simulink model "VLI_OLC_sim"  (R2023a)
settings: Solver=VariableStepAuto  StartTime=0.0  StopTime=1000  RelTol=1e-3
values from neighbouring files (symbols this model uses):
  E = diag([0.95, 0.95, 0.95])    [VLI_OLC_parameter.m]
  J0 = [20, 2, 0.9; 2, 17, 0.5; 0.9, 0.5, 15]    [VLI_OLC_parameter.m]
  k2 = 1    [VLI_OLC_parameter.m]
  k3 = 2    [VLI_OLC_parameter.m]
  Q0 = [-0.2, 0.3, -0.2]    [VLI_OLC_parameter.m]
  Q00 = sqrt(0.83)    [VLI_OLC_parameter.m]
  sig = 1    [VLI_OLC_parameter.m]
  td = 0.01    [VLI_OLC_parameter.m]
  tor = 0.01    [VLI_OLC_parameter.m]
  torque0 = 0.001    [VLI_OLC_parameter.m]
  Tu = 0.03    [VLI_OLC_parameter.m]
  Tv = 0.03    [VLI_OLC_parameter.m]
  w0 = [0, 0, 0]'    [VLI_OLC_parameter.m]
libraries: matrix_library x3, sharedutil x1
settings Model: Creator=bin.lu  LastModifiedBy=bin.lu
settings DataIOCC: ReturnWorkspaceOutputs=off  TimeSaveName=t1

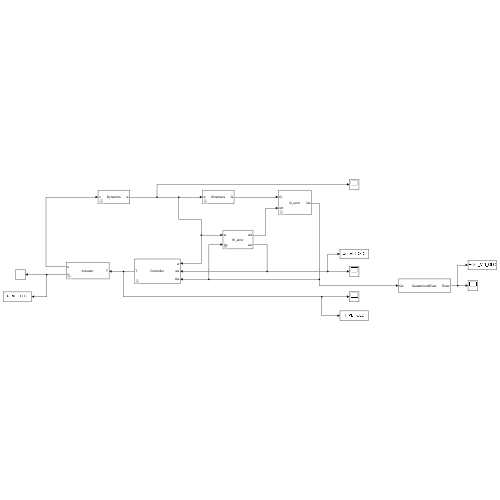
[thumbnail: Simulink's stored preview of the top-level diagram]
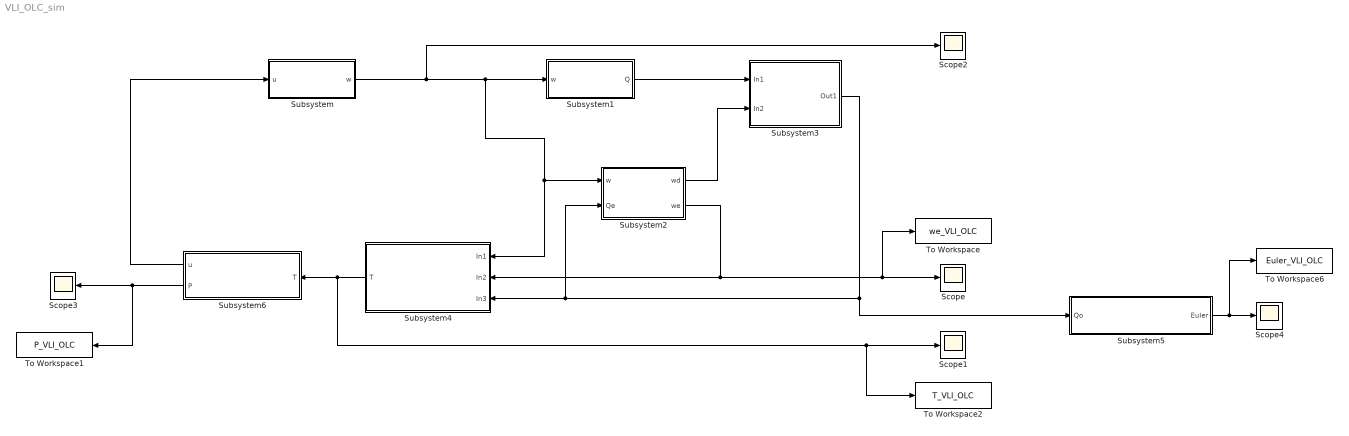
== system VLI_OLC_sim ==
  Scope{,1..4} (5 alike) : Scope
  Subsystem : Subsystem
      mask DialogControl ParameterGroupVar Prompt: 参数
      mask Display:
      | disp('Dynamics');
      | port_label('input', 1, 'u');
      | port_label('output', 1, 'w');
  Subsystem1 : Subsystem
      mask DialogControl ParameterGroupVar Prompt: 参数
      mask Display:
      | disp('Kinemacs');
      | port_label('input', 1, 'w');
      | port_label('output', 1, 'Q');
  Subsystem2 : Subsystem
      mask DialogControl ParameterGroupVar Prompt: 参数
      mask Display:
      | disp('W_error');
      | port_label('input', 1, 'w');
      | port_label('input', 2, 'Qe');
      | port_label('output', 2, 'we');
      | port_label('output', 1, 'wd');
  Subsystem3 : Subsystem
      mask DialogControl ParameterGroupVar Prompt: 参数
      mask Display:
      | disp('Q_error');
      | port_label('input', 1, 'Q');
      | port_label('input', 2, 'wd');
      | port_label('output', 1, 'Qe');
  Subsystem4 : Subsystem
      mask DialogControl ParameterGroupVar Prompt: 参数
      mask Display:
      | disp('Controller');
      | port_label('input', 1, 'w');
      | port_label('input', 2, 'we');
      | port_label('input', 3, 'Qe');
      | port_label('output', 1, 'T');
  Subsystem5 : Subsystem
      mask Display:
      | disp('Quaternion2Euler')
      | port_label('input', 1, 'Qo')
      | port_label('output', 1, 'Euler')
  Subsystem6 : Subsystem
      mask DialogControl ParameterGroupVar Prompt: 参数
      mask Display:
      | disp('Actuator');
      | port_label('input', 1, 'T');
      | port_label('output', 1, 'u');
      | port_label('output', 2, 'P');
  To Workspace : ToWorkspace  VariableName=we_VLI_OLC  SampleTime=-1
      settings: Save2DSignal=2-D array (concatenate along first dimension)
  To Workspace1 : ToWorkspace  VariableName=P_VLI_OLC  SampleTime=0.01
  To Workspace2 : ToWorkspace  VariableName=T_VLI_OLC  SampleTime=-1
      settings: Save2DSignal=2-D array (concatenate along first dimension)
  To Workspace6 : ToWorkspace  VariableName=Euler_VLI_OLC  SampleTime=-1
      settings: Save2DSignal=2-D array (concatenate along first dimension)
  wires:
  Subsystem2/1(wd) -> Subsystem3/2(In2)
  Subsystem3/1(Out1) -> Subsystem5/1(Qo), Subsystem2/2(Qe), Subsystem4/3(In3)
  Subsystem6/2(P) -> To Workspace1/1, Scope3/1
  Subsystem2/2(we) -> Subsystem4/2(In2), To Workspace/1, Scope/1
  Subsystem4/1(T) -> To Workspace2/1, Scope1/1, Subsystem6/1(T)
  Subsystem6/1(u) -> Subsystem/1(u)
  Subsystem1/1(Q) -> Subsystem3/1(In1)
  Subsystem/1(w) -> Subsystem1/1(w), Subsystem4/1(In1), Subsystem2/1(w), Scope2/1
  Subsystem5/1(Euler) -> To Workspace6/1, Scope4/1

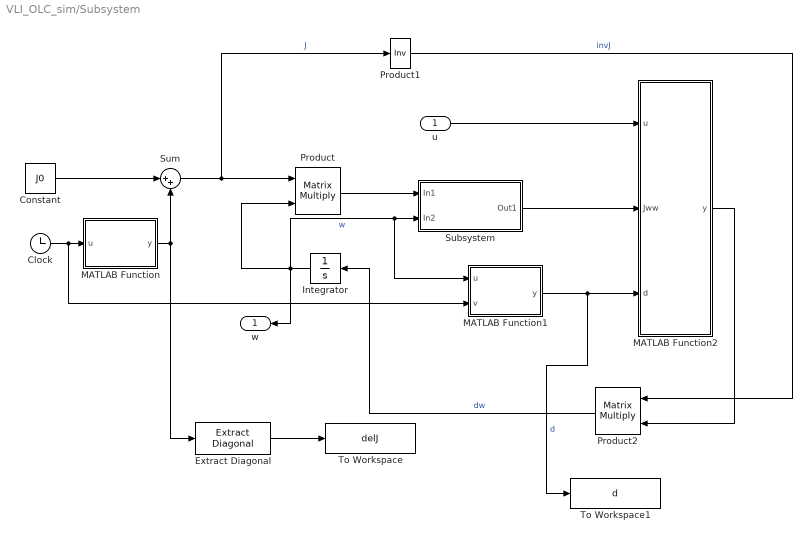
== system VLI_OLC_sim/Subsystem ==
  u : Inport
  Clock : Clock
  Constant : Constant  Value=J0
  Extract Diagonal : matrix_library/Extract Diagonal
      settings: LibrarySourceBlock=|
      | simulink/Matrix
      | Operations/Extract Diagonal
  Integrator : Integrator  InitialCondition=w0
  MATLAB Function : MATLAB Function  TreatAsAtomicUnit=on
  MATLAB Function1 : MATLAB Function  TreatAsAtomicUnit=on
  MATLAB Function2 : MATLAB Function  TreatAsAtomicUnit=on
  Product : Product  Multiplication=Matrix(*)
  Product1 : Product  Inputs=/  Multiplication=Matrix(*)
  Product2 : Product  Multiplication=Matrix(*)
  Subsystem : Subsystem
      mask Display:
      | disp('Cross \nProduct')
      | port_label('input', 1, 'X')
      | port_label('input', 2, 'Y')
      | port_label('output', 1, 'X*Y')
  Sum : Sum  Inputs=|++
  To Workspace : ToWorkspace  VariableName=delJ  SampleTime=-1
      settings: Save2DSignal=2-D array (concatenate along first dimension)
  To Workspace1 : ToWorkspace  VariableName=d  SampleTime=-1
      settings: Save2DSignal=2-D array (concatenate along first dimension)
  w : Outport
  wires:
  MATLAB Function/1(y) -> Extract Diagonal/1, Sum/2
  Constant/1 -> Sum/1
  Clock/1 -> MATLAB Function1/2(v), MATLAB Function/1(u)
  Sum/1 -> Product1/1, Product/1  "J"
  Integrator/1 -> w/1, MATLAB Function1/1(u), Subsystem/2(In2), Product/2  "w"
  Product/1 -> Subsystem/1(In1)
  Subsystem/1(Out1) -> MATLAB Function2/2(Jww)
  Product2/1 -> Integrator/1  "dw"
  MATLAB Function1/1(y) -> To Workspace1/1, MATLAB Function2/3(d)  "d"
  u/1 -> MATLAB Function2/1(u)
  MATLAB Function2/1(y) -> Product2/2
  Product1/1 -> Product2/1  "invJ"
  Extract Diagonal/1 -> To Workspace/1

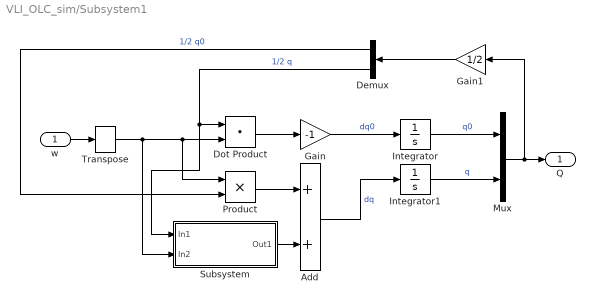
== system VLI_OLC_sim/Subsystem1 ==
  w : Inport
  Add : Sum
  Demux : Demux  Outputs=[1 3]
  Dot Product : DotProduct  OutDataTypeStr=Inherit: Inherit via internal rule
  Gain : Gain  Gain=-1
  Gain1 : Gain  Gain=1/2
  Integrator : Integrator  InitialCondition=Q00
  Integrator1 : Integrator  InitialCondition=Q0
  Mux : Mux  Inputs=[1 3]
  Product : Product
  Subsystem : Subsystem
      mask Display:
      | disp('Cross \nProduct')
      | port_label('input', 1, 'X')
      | port_label('input', 2, 'Y')
      | port_label('output', 1, 'X*Y')
  Transpose : matrix_library/Transpose
  Q : Outport
  wires:
  Dot Product/1 -> Gain/1
  w/1 -> Transpose/1
  Add/1 -> Integrator1/1  "dq"
  Demux/2 -> Subsystem/1(In1), Dot Product/1  "1/2 q"
  Integrator1/1 -> Mux/2  "q"
  Product/1 -> Add/1
  Gain/1 -> Integrator/1  "dq0"
  Integrator/1 -> Mux/1  "q0"
  Mux/1 -> Gain1/1, Q/1
  Gain1/1 -> Demux/1
  Subsystem/1(Out1) -> Add/2
  Demux/1 -> Product/2  "1/2 q0"
  Transpose/1 -> Subsystem/2(In2), Product/1, Dot Product/2

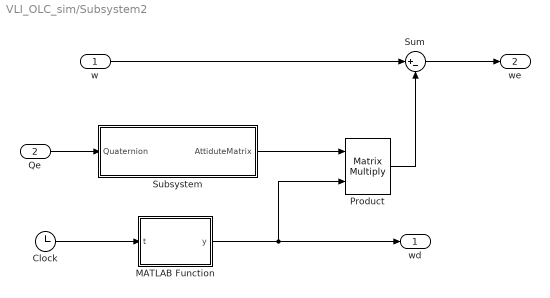
== system VLI_OLC_sim/Subsystem2 ==
  w : Inport
  Qe : Inport  Port=2
  Clock : Clock
  MATLAB Function : MATLAB Function  TreatAsAtomicUnit=on
  Product : Product  Multiplication=Matrix(*)
  Subsystem : Subsystem
      mask Display:
      | disp('Quaternion2 \nAttitudeMatrix')
      | port_label('input', 1, 'Qua')
      | port_label('output', 1, 'Matrix')
  Sum : Sum  Inputs=|+-
  wd : Outport
  we : Outport  Port=2
  wires:
  Qe/1 -> Subsystem/1(Quaternion)
  Clock/1 -> MATLAB Function/1(t)
  Subsystem/1(AttiduteMatrix) -> Product/1
  MATLAB Function/1(y) -> wd/1, Product/2
  w/1 -> Sum/1
  Sum/1 -> we/1
  Product/1 -> Sum/2

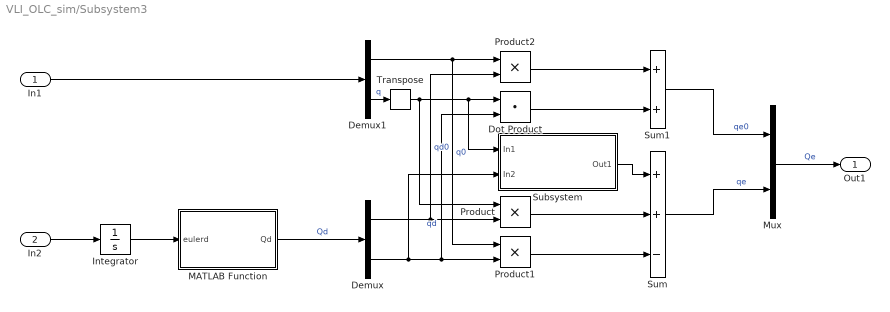
== system VLI_OLC_sim/Subsystem3 ==
  In1 : Inport
  In2 : Inport  Port=2
  Demux : Demux  Outputs=[1 3]
  Demux1 : Demux  Outputs=[1 3]
  Dot Product : DotProduct  OutDataTypeStr=Inherit: Inherit via internal rule
  Integrator : Integrator
  MATLAB Function : MATLAB Function  TreatAsAtomicUnit=on
  Mux : Mux  Inputs=[1 3]
  Product : Product
  Product1 : Product
  Product2 : Product
  Subsystem : Subsystem
      mask Display:
      | disp('Cross \nProduct')
      | port_label('input', 1, 'X')
      | port_label('input', 2, 'Y')
      | port_label('output', 1, 'X*Y')
  Sum : Sum  Inputs=++-
  Sum1 : Sum
  Transpose : matrix_library/Transpose
  Out1 : Outport
  wires:
  In2/1 -> Integrator/1
  Integrator/1 -> MATLAB Function/1(eulerd)
  MATLAB Function/1(Qd) -> Demux/1  "Qd"
  In1/1 -> Demux1/1
  Demux/1 -> Product2/2, Product/2  "qd0"
  Demux1/2 -> Transpose/1  "q"
  Demux/2 -> Subsystem/2(In2), Dot Product/2, Product1/2  "qd"
  Demux1/1 -> Product2/1, Product1/1  "q0"
  Subsystem/1(Out1) -> Sum/1
  Product/1 -> Sum/2
  Product1/1 -> Sum/3
  Product2/1 -> Sum1/1
  Dot Product/1 -> Sum1/2
  Sum1/1 -> Mux/1  "qe0"
  Sum/1 -> Mux/2  "qe"
  Mux/1 -> Out1/1  "Qe"
  Transpose/1 -> Product/1, Subsystem/1(In1), Dot Product/1

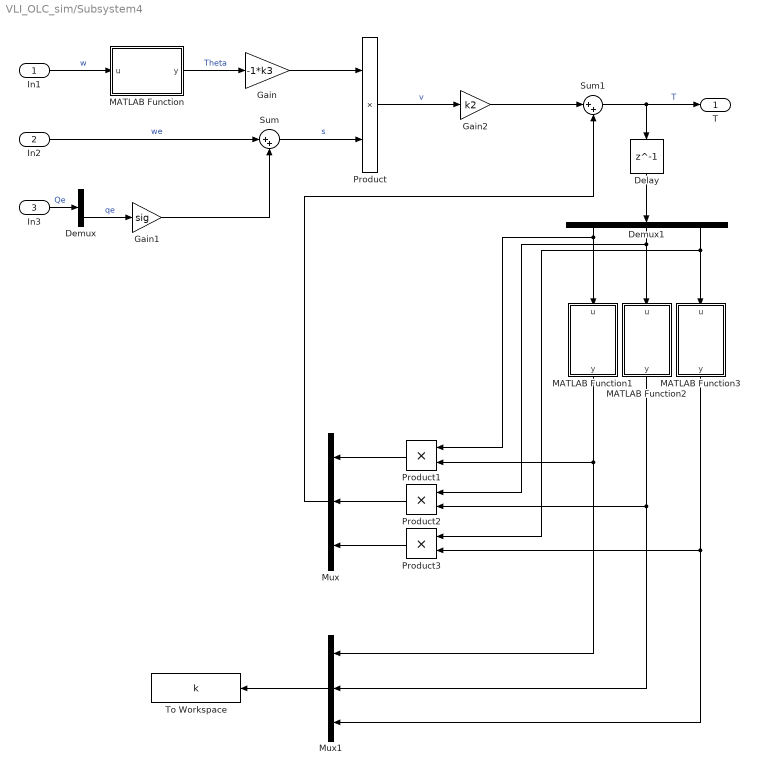
== system VLI_OLC_sim/Subsystem4 ==
  In1 : Inport
  In2 : Inport  Port=2
  In3 : Inport  Port=3
  Delay : Delay  DelayLength=1  InitialCondition=0  SampleTime=tor
  Demux : Demux  Outputs=[1 3]
  Demux1 : Demux  Outputs=[1 1 1]
  Gain : Gain  Gain=-1*k3
  Gain1 : Gain  Gain=sig
  Gain2 : Gain  Gain=k2
  MATLAB Function : MATLAB Function  TreatAsAtomicUnit=on
  MATLAB Function1 : MATLAB Function  TreatAsAtomicUnit=on
  MATLAB Function2 : MATLAB Function  TreatAsAtomicUnit=on
  MATLAB Function3 : MATLAB Function  TreatAsAtomicUnit=on
  Mux : Mux  Inputs=[1 1 1]
  Mux1 : Mux  Inputs=[1 1 1]
  Product{,1..3} (4 alike) : Product
  Sum : Sum  Inputs=|++
  Sum1 : Sum  Inputs=|++
  To Workspace : ToWorkspace  VariableName=k  SampleTime=-1
      settings: Save2DSignal=2-D array (concatenate along first dimension)
  T : Outport
  wires:
  In1/1 -> MATLAB Function/1(u)  "w"
  MATLAB Function/1(y) -> Gain/1  "Theta"
  In3/1 -> Demux/1  "Qe"
  In2/1 -> Sum/1  "we"
  Gain1/1 -> Sum/2
  Gain/1 -> Product/1
  Sum/1 -> Product/2  "s"
  Product/1 -> Gain2/1  "v"
  Gain2/1 -> Sum1/1
  Sum1/1 -> T/1, Delay/1  "T"
  Demux/2 -> Gain1/1  "qe"
  Delay/1 -> Demux1/1
  Demux1/1 -> MATLAB Function1/1(u), Product1/1
  Demux1/2 -> MATLAB Function2/1(u), Product2/1
  Demux1/3 -> MATLAB Function3/1(u), Product3/1
  MATLAB Function1/1(y) -> Mux1/1, Product1/2
  MATLAB Function2/1(y) -> Mux1/2, Product2/2
  MATLAB Function3/1(y) -> Mux1/3, Product3/2
  Product2/1 -> Mux/2
  Product1/1 -> Mux/1
  Product3/1 -> Mux/3
  Mux/1 -> Sum1/2
  Mux1/1 -> To Workspace/1

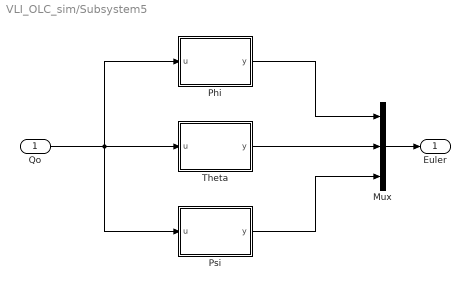
== system VLI_OLC_sim/Subsystem5 ==
  Qo : Inport
  Mux : Mux  Inputs=3
  Phi : MATLAB Function  TreatAsAtomicUnit=on
  Psi : MATLAB Function  TreatAsAtomicUnit=on
  Theta : MATLAB Function  TreatAsAtomicUnit=on
  Euler : Outport
  wires:
  Mux/1 -> Euler/1
  Theta/1(y) -> Mux/2
  Phi/1(y) -> Mux/1
  Psi/1(y) -> Mux/3
  Qo/1 -> Psi/1(u), Phi/1(u), Theta/1(u)

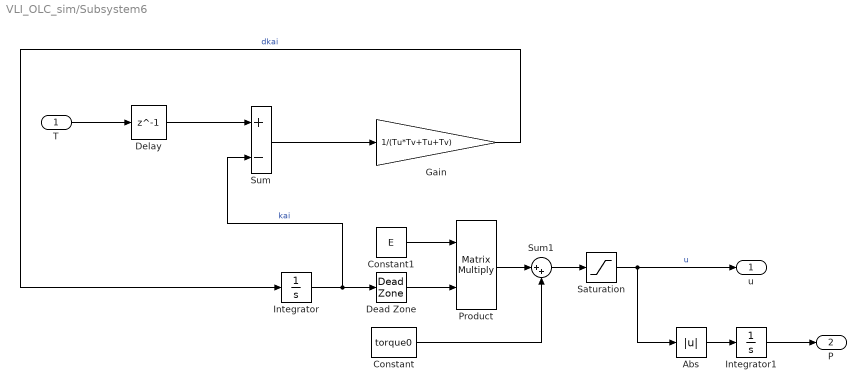
== system VLI_OLC_sim/Subsystem6 ==
  T : Inport
  Abs : Abs  SaturateOnIntegerOverflow=off
  Constant : Constant  Value=torque0
  Constant1 : Constant  Value=E
  Dead Zone : DeadZone  LowerValue=-0.001  UpperValue=0.001
  Delay : Delay  DelayLength=1  InitialCondition=0  SampleTime=td
  Gain : Gain  Gain=1/(Tu*Tv+Tu+Tv)
  Integrator : Integrator
  Integrator1 : Integrator
  Product : Product  Multiplication=Matrix(*)
  Saturation : Saturate  UpperLimit=1  LowerLimit=-1
  Sum : Sum  Inputs=+-
  Sum1 : Sum  Inputs=|++
  u : Outport
  P : Outport  Port=2
  wires:
  T/1 -> Delay/1
  Integrator/1 -> Sum/2, Dead Zone/1  "kai"
  Saturation/1 -> Abs/1, u/1  "u"
  Delay/1 -> Sum/1
  Sum/1 -> Gain/1
  Gain/1 -> Integrator/1  "dkai"
  Constant1/1 -> Product/1
  Integrator1/1 -> P/1
  Dead Zone/1 -> Product/2
  Product/1 -> Sum1/1
  Sum1/1 -> Saturation/1
  Constant/1 -> Sum1/2
  Abs/1 -> Integrator1/1

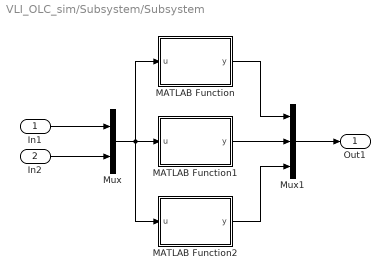
== system VLI_OLC_sim/Subsystem/Subsystem ==
  In1 : Inport
  In2 : Inport  Port=2
  MATLAB Function : MATLAB Function  TreatAsAtomicUnit=on
  MATLAB Function1 : MATLAB Function  TreatAsAtomicUnit=on
  MATLAB Function2 : MATLAB Function  TreatAsAtomicUnit=on
  Mux : Mux  Inputs=[3 3]
  Mux1 : Mux  Inputs=[1 1 1]
  Out1 : Outport
  wires:
  In1/1 -> Mux/1
  In2/1 -> Mux/2
  Mux/1 -> MATLAB Function2/1(u), MATLAB Function/1(u), MATLAB Function1/1(u)
  MATLAB Function/1(y) -> Mux1/1
  MATLAB Function1/1(y) -> Mux1/2
  MATLAB Function2/1(y) -> Mux1/3
  Mux1/1 -> Out1/1

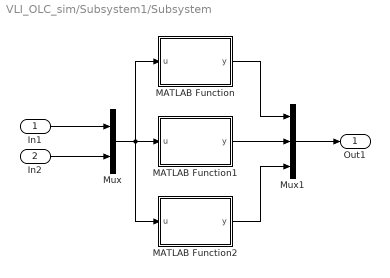
== system VLI_OLC_sim/Subsystem1/Subsystem ==
  In1 : Inport
  In2 : Inport  Port=2
  MATLAB Function : MATLAB Function  TreatAsAtomicUnit=on
  MATLAB Function1 : MATLAB Function  TreatAsAtomicUnit=on
  MATLAB Function2 : MATLAB Function  TreatAsAtomicUnit=on
  Mux : Mux  Inputs=[3 3]
  Mux1 : Mux  Inputs=[1 1 1]
  Out1 : Outport
  wires:
  In1/1 -> Mux/1
  In2/1 -> Mux/2
  Mux/1 -> MATLAB Function2/1(u), MATLAB Function/1(u), MATLAB Function1/1(u)
  MATLAB Function/1(y) -> Mux1/1
  MATLAB Function1/1(y) -> Mux1/2
  MATLAB Function2/1(y) -> Mux1/3
  Mux1/1 -> Out1/1

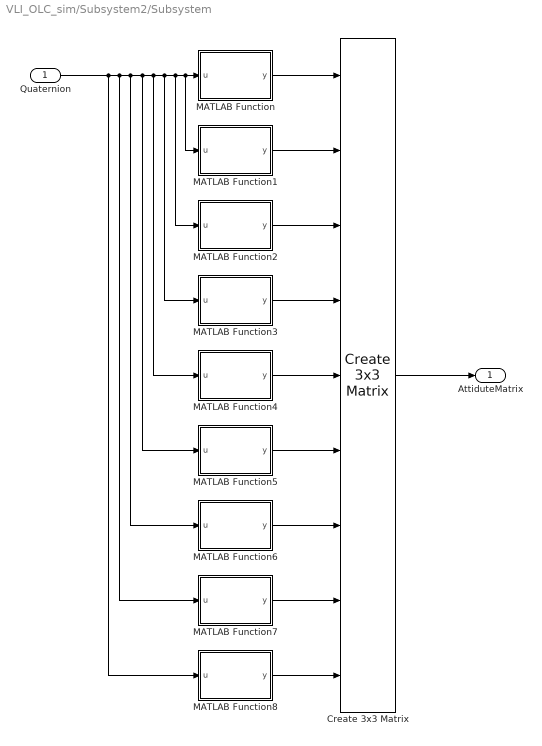
== system VLI_OLC_sim/Subsystem2/Subsystem ==
  Quaternion : Inport
  Create 3x3 Matrix : sharedutil/Create 3x3 Matrix  aMode=aMode
  MATLAB Function : MATLAB Function  TreatAsAtomicUnit=on
  MATLAB Function1 : MATLAB Function  TreatAsAtomicUnit=on
  MATLAB Function2 : MATLAB Function  TreatAsAtomicUnit=on
  MATLAB Function3 : MATLAB Function  TreatAsAtomicUnit=on
  MATLAB Function4 : MATLAB Function  TreatAsAtomicUnit=on
  MATLAB Function5 : MATLAB Function  TreatAsAtomicUnit=on
  MATLAB Function6 : MATLAB Function  TreatAsAtomicUnit=on
  MATLAB Function7 : MATLAB Function  TreatAsAtomicUnit=on
  MATLAB Function8 : MATLAB Function  TreatAsAtomicUnit=on
  AttiduteMatrix : Outport
  wires:
  Create 3x3 Matrix/1 -> AttiduteMatrix/1
  Quaternion/1 -> MATLAB Function8/1(u), MATLAB Function7/1(u), MATLAB Function6/1(u), MATLAB Function5/1(u), MATLAB Function4/1(u), MATLAB Function3/1(u), MATLAB Function2/1(u), MATLAB Function1/1(u), MATLAB Function/1(u)
  MATLAB Function/1(y) -> Create 3x3 Matrix/1
  MATLAB Function1/1(y) -> Create 3x3 Matrix/2
  MATLAB Function2/1(y) -> Create 3x3 Matrix/3
  MATLAB Function3/1(y) -> Create 3x3 Matrix/4
  MATLAB Function4/1(y) -> Create 3x3 Matrix/5
  MATLAB Function5/1(y) -> Create 3x3 Matrix/6
  MATLAB Function6/1(y) -> Create 3x3 Matrix/7
  MATLAB Function7/1(y) -> Create 3x3 Matrix/8
  MATLAB Function8/1(y) -> Create 3x3 Matrix/9

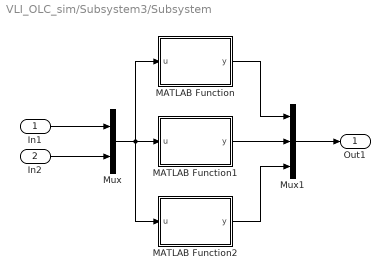
== system VLI_OLC_sim/Subsystem3/Subsystem ==
  In1 : Inport
  In2 : Inport  Port=2
  MATLAB Function : MATLAB Function  TreatAsAtomicUnit=on
  MATLAB Function1 : MATLAB Function  TreatAsAtomicUnit=on
  MATLAB Function2 : MATLAB Function  TreatAsAtomicUnit=on
  Mux : Mux  Inputs=[3 3]
  Mux1 : Mux  Inputs=[1 1 1]
  Out1 : Outport
  wires:
  In1/1 -> Mux/1
  In2/1 -> Mux/2
  Mux/1 -> MATLAB Function2/1(u), MATLAB Function/1(u), MATLAB Function1/1(u)
  MATLAB Function/1(y) -> Mux1/1
  MATLAB Function1/1(y) -> Mux1/2
  MATLAB Function2/1(y) -> Mux1/3
  Mux1/1 -> Out1/1

== matlab function VLI_OLC_sim/Subsystem2/Subsystem/MATLAB Function ==
  data: u input; y output
function y = fcn(u)

y = 1 - 2*(u(3)*u(3) + u(4)*u(4));

== matlab function VLI_OLC_sim/Subsystem2/Subsystem/MATLAB Function1 ==
  data: u input; y output
function y = fcn(u)

y = 2*(u(2)*u(3) + u(1)*u(4));

== matlab function VLI_OLC_sim/Subsystem2/Subsystem/MATLAB Function2 ==
  data: u input; y output
function y = fcn(u)

y = 2*(-u(1)*u(3) + u(2)*u(4));

== matlab function VLI_OLC_sim/Subsystem2/Subsystem/MATLAB Function3 ==
  data: u input; y output
function y = fcn(u)

y = 2*(u(2)*u(3) - u(1)*u(4));

== matlab function VLI_OLC_sim/Subsystem2/Subsystem/MATLAB Function4 ==
  data: u input; y output
function y = fcn(u)

y = 1 - 2*(u(2)*u(2) + u(4)*u(4));

== matlab function VLI_OLC_sim/Subsystem2/Subsystem/MATLAB Function5 ==
  data: u input; y output
function y = fcn(u)

y = 2*(u(1)*u(2) + u(3)*u(4));

== matlab function VLI_OLC_sim/Subsystem2/Subsystem/MATLAB Function6 ==
  data: u input; y output
function y = fcn(u)

y = 2*(u(1)*u(3) + u(2)*u(4));

== matlab function VLI_OLC_sim/Subsystem2/Subsystem/MATLAB Function7 ==
  data: u input; y output
function y = fcn(u)

y = 2*(-u(1)*u(2) + u(3)*u(4));

== matlab function VLI_OLC_sim/Subsystem2/Subsystem/MATLAB Function8 ==
  data: u input; y output
function y = fcn(u)

y = 1 - 2*(u(2)*u(2) + u(3)*u(3));

== matlab function VLI_OLC_sim/Subsystem5/Theta ==
  data: u input; y output
function y = fcn(u)

y = asin(-2*(u(2)*u(4) - u(1)*u(3)));

== matlab function VLI_OLC_sim/Subsystem3/MATLAB Function ==
  data: eulerd input; Qd output
function Qd = fcn(eulerd)

Qd = zeros(4,1);
Qd(1) = cos(eulerd(1)/2)*cos(eulerd(2)/2)*cos(eulerd(3)/2) + sin(eulerd(1)/2)*sin(eulerd(2)/2)*sin(eulerd(3)/2);
Qd(2) = sin(eulerd(1)/2)*cos(eulerd(2)/2)*cos(eulerd(3)/2) - cos(eulerd(1)/2)*sin(eulerd(2)/2)*sin(eulerd(3)/2);
Qd(3) = cos(eulerd(1)/2)*sin(eulerd(2)/2)*cos(eulerd(3)/2) + sin(eulerd(1)/2)*cos(eulerd(2)/2)*sin(eulerd(3)/2);
Qd(4) = -sin(eulerd(1)/2)*sin(eulerd(2)/2)*cos(eulerd(3)/2) + cos(eulerd(1)/2)*cos(eulerd(2)/2)*sin(eulerd(3)/2);

== matlab function VLI_OLC_sim/Subsystem3/Subsystem/MATLAB Function ==
  data: u input; y output
function y = fcn(u)

y = u(2)*u(6) - u(3)*u(5);

== matlab function VLI_OLC_sim/Subsystem3/Subsystem/MATLAB Function1 ==
  data: u input; y output
function y = fcn(u)

y = u(3)*u(4) - u(1)*u(6);

== matlab function VLI_OLC_sim/Subsystem3/Subsystem/MATLAB Function2 ==
  data: u input; y output
function y = fcn(u)

y = u(1)*u(5) - u(2)*u(4);

== matlab function VLI_OLC_sim/Subsystem4/MATLAB Function ==
  data: u input; y output
function y = fcn(u)

w = [u(1); u(2); u(3)];
y = (norm(w))^2+norm(w)+1;

== matlab function VLI_OLC_sim/Subsystem4/MATLAB Function1 ==
  data: u input; y output
function y = fcn(u)

r1 = 4;
r2 = 2;
epsi = 0.1;
y = exp(-r1*(norm(u)+epsi)^r2);

== matlab function VLI_OLC_sim/Subsystem4/MATLAB Function2 ==
  data: u input; y output
function y = fcn(u)

r1 = 4;
r2 = 2;
epsi = 0.1;
y = exp(-r1*(norm(u)+epsi)^r2);

== matlab function VLI_OLC_sim/Subsystem4/MATLAB Function3 ==
  data: u input; y output
function y = fcn(u)

r1 = 4;
r2 = 2;
epsi = 0.1;
y = exp(-r1*(norm(u)+epsi)^r2);

== matlab function VLI_OLC_sim/Subsystem5/Psi ==
  data: u input; y output
function y = fcn(u)

y = atan(2*(u(2)*u(3) + u(1)*u(4))/(u(1)^2 + u(2)^2 - u(3)^2 - u(4)^2));

== matlab function VLI_OLC_sim/Subsystem/MATLAB Function ==
  data: u input; y output
function y = fcn(u)

y = [(3+sin(0.5*u))*exp(-0.1*u)+1, 0, 0; 0, (4+sin(0.5*u))*exp(-0.1*u)+2, 0; 0, 0, (5+sin(0.5*u))*exp(-0.1*u)-1];

== matlab function VLI_OLC_sim/Subsystem/MATLAB Function1 ==
  data: u input; y output; v input
function y = fcn(u,v)

phi = 0.5+norm(u);
y = [-3*cos(phi*v)-6*sin(0.3*phi*v)+3; 1.5*sin(phi*v)-3*cos(0.5*phi*v)-2; -3*sin(phi*v)+8*sin(0.4*phi*v)-1]*0.001;

== matlab function VLI_OLC_sim/Subsystem/MATLAB Function2 ==
  data: u input; y output; Jww input; d input
function y = fcn(u, Jww, d)

y = zeros(3, 1);
y(1) = u(1)+Jww(1)+d(1);
y(2) = u(2)+Jww(2)+d(2);
y(3) = u(3)+Jww(3)+d(3);

== matlab function VLI_OLC_sim/Subsystem/Subsystem/MATLAB Function ==
  data: u input; y output
function y = fcn(u)

y = u(2)*u(6) - u(3)*u(5);

== matlab function VLI_OLC_sim/Subsystem/Subsystem/MATLAB Function1 ==
  data: u input; y output
function y = fcn(u)

y = u(3)*u(4) - u(1)*u(6);

== matlab function VLI_OLC_sim/Subsystem/Subsystem/MATLAB Function2 ==
  data: u input; y output
function y = fcn(u)

y = u(1)*u(5) - u(2)*u(4);

== matlab function VLI_OLC_sim/Subsystem1/Subsystem/MATLAB Function ==
  data: u input; y output
function y = fcn(u)

y = u(2)*u(6) - u(3)*u(5);

== matlab function VLI_OLC_sim/Subsystem1/Subsystem/MATLAB Function1 ==
  data: u input; y output
function y = fcn(u)

y = u(3)*u(4) - u(1)*u(6);

== matlab function VLI_OLC_sim/Subsystem1/Subsystem/MATLAB Function2 ==
  data: u input; y output
function y = fcn(u)

y = u(1)*u(5) - u(2)*u(4);

== matlab function VLI_OLC_sim/Subsystem5/Phi ==
  data: u input; y output
function y = fcn(u)

y = atan(2*(u(1)*u(2) + u(3)*u(4))/(u(1)^2 - u(2)^2 - u(3)^2 + u(4)^2));

== matlab function VLI_OLC_sim/Subsystem2/MATLAB Function ==
  data: t input; y output
function y = fcn(t)

psi = 0.1*t;
y = [cos(psi); -sin(psi); -cos(psi)]*0.01;
